simulink model "zadanie3"  (R2020b)
settings: Solver=FixedStepDiscrete  StartTime=0.0  StopTime=0  RelTol=1e-3
libraries: CPOiS_SourcesSinks x5, CPOiS_DataManipulation x3, CPOiS_General x1
settings Model: Creator=jrybarz  LastModifiedBy=jrybarz

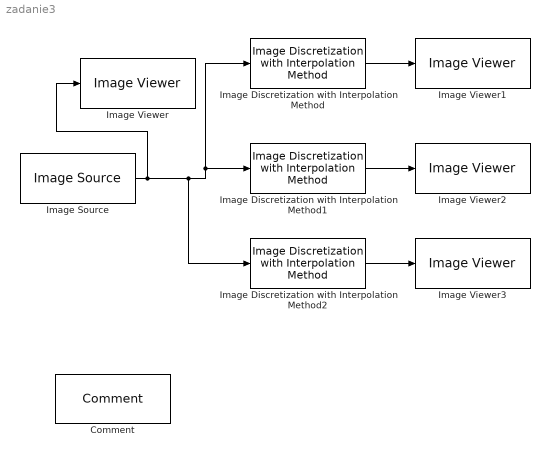
== system zadanie3 ==
  Comment : CPOiS_General/Comment
      settings: SourceProductName=CPOiS - Digital image and signal processing
  Image Discretization with Interpolation Method : CPOiS_DataManipulation/Image Discretization with Interpolation Method  factor=5  method=nearest
      settings: SourceProductName=CPOiS - Digital image and signal processing
  Image Discretization with Interpolation Method1 : CPOiS_DataManipulation/Image Discretization with Interpolation Method  factor=5  method=bilinear
      settings: SourceProductName=CPOiS - Digital image and signal processing
  Image Discretization with Interpolation Method2 : CPOiS_DataManipulation/Image Discretization with Interpolation Method  factor=5  method=bicubic
      settings: SourceProductName=CPOiS - Digital image and signal processing
  Image Source : CPOiS_SourcesSinks/Image Source  FileSelection=printedtext.png
      settings: SourceProductName=CPOiS - Digital image and signal processing
  Image Viewer{,1..3} (4 alike) : CPOiS_SourcesSinks/Image Viewer
      settings: SourceProductName=CPOiS - Digital image and signal processing
  wires:
  Image Source/1 -> Image Viewer/1, Image Discretization with Interpolation Method2/1, Image Discretization with Interpolation Method1/1, Image Discretization with Interpolation Method/1
  Image Discretization with Interpolation Method2/1 -> Image Viewer3/1
  Image Discretization with Interpolation Method1/1 -> Image Viewer2/1
  Image Discretization with Interpolation Method/1 -> Image Viewer1/1
